simulink model "main_indi"  (R2018a)
settings: Solver=VariableStepAuto  StartTime=0.0  StopTime=inf  RelTol=1e-3
InitFcn:
  | G1_inverse;
undefined symbols (not defined in the file): G1_inv
libraries: aerolibutil x4, shared6dof x1, vrlib x1, simulink x1, powerlib_meascontrol x1, aerolibanimutils x1, aerolibnav x1
settings Model: Creator=PSere  LastModifiedBy=PSere

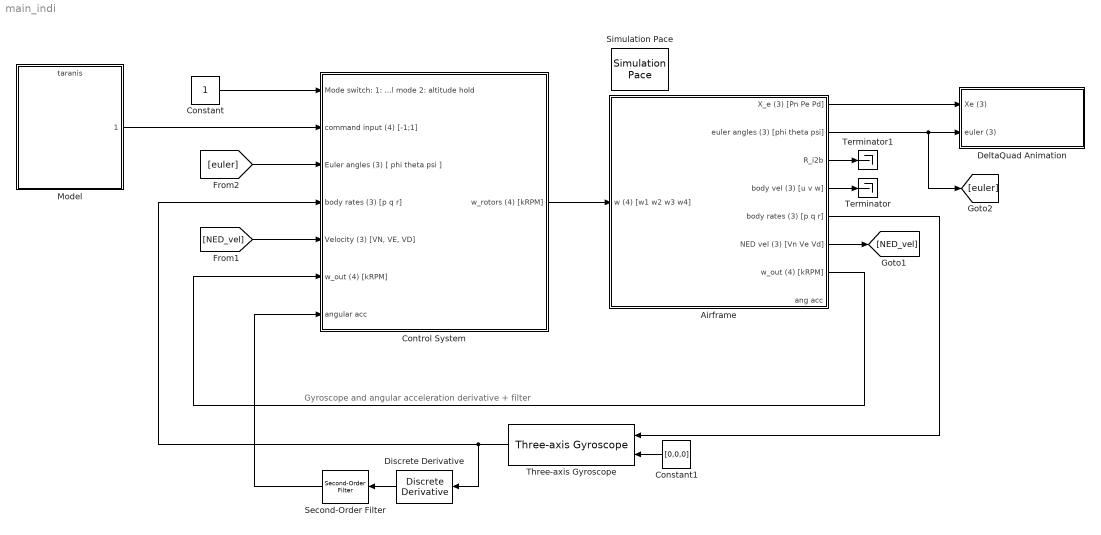
== system main_indi ==
  note: Gyroscope and angular acceleration derivative + filter
  Airframe : Subsystem
  Constant : Constant
  Constant1 : Constant  Value=[0,0,0]
  Control System : Subsystem
  DeltaQuad Animation : Subsystem
  Discrete Derivative : simulink/Discrete/Discrete Derivative  gainval=1.0  ICPrevScaledInput=0.0  OutMin=[]  OutMax=[]  OutDataType=fixdt(1, 16)  OutScaling=2^-10  DoSatur=off
  Model : ModelReference  ModelNameDialog=taranis.mdl  SimulationMode=Normal  ModelReferenceVersion=1.8
  Second-Order Filter : powerlib_meascontrol/Filters/Second-Order Filter  FilterType=Lowpass  Fo=2  Zeta=1  Ts=0  Initialize=on  Vac_Init="[0,  0,  60]"  Vdc_Init=0  PlotResponse=off  FreqRange=[0, 500, 1]
      settings: SourceProductName=Simscape Power Systems  SourceProductBaseCode=PS
  Simulation Pace : aerolibanimutils/Simulation Pace  SimulationPace=1  SleepMode=MATLAB Thread  OutputPaceError=off  SampleTime=1/30
  Terminator : Terminator
  Terminator1 : Terminator
  Three-axis Gyroscope : aerolibnav/Three-axis Gyroscope  dtype_g=on  w_g=190  z_g=0.707  g_sf_cc=[1 0 0; 0 1 0; 0 0 1]  g_bias=[0 0 0]  g_sen=[0 0 0]  g_Ts=0  g_rand=on  g_seeds=[23093 23094 23095]  g_pow=[0.0001 0.0001 0.0001]  g_sat="[-inf  -inf  -inf  inf inf inf]"
      settings: SourceProductName=Aerospace Blockset  SourceProductBaseCode=AE
  wires:
  Model/1 -> Control System/2(command input (4) [-1;1])
  Control System/1(w_rotors (4) [kRPM]) -> Airframe/1(w (4) [w1 w2 w3 w4])
  Airframe/1(X_e (3) [Pn Pe Pd]) -> DeltaQuad Animation/1(Xe (3))
  Airframe/4(body vel (3) [u v w]) -> Terminator/1
  Airframe/2(euler angles (3) [phi theta psi]) -> [euler], DeltaQuad Animation/2(euler (3))
  Airframe/3(R_i2b) -> Terminator1/1
  Constant/1 -> Control System/1(Mode switch: 1: manual mode 2: altitude hold)
  Airframe/5(body rates (3) [p q r]) -> Three-axis Gyroscope/1
  Airframe/6("NED vel (3) [Vn Ve Vd] ") -> [NED_vel]
  [NED_vel] -> Control System/5("Velocity (3) [VN, VE, VD]")
  Three-axis Gyroscope/1 -> Discrete Derivative/1, Control System/4(body rates (3) [p q r])
  [euler] -> Control System/3(Euler angles (3) [ phi theta psi ])
  Airframe/7(w_out (4) [kRPM]) -> Control System/6(w_out (4) [kRPM])
  Constant1/1 -> Three-axis Gyroscope/2
  Discrete Derivative/1 -> Second-Order Filter/1
  Second-Order Filter/1 -> Control System/7(angular acc)

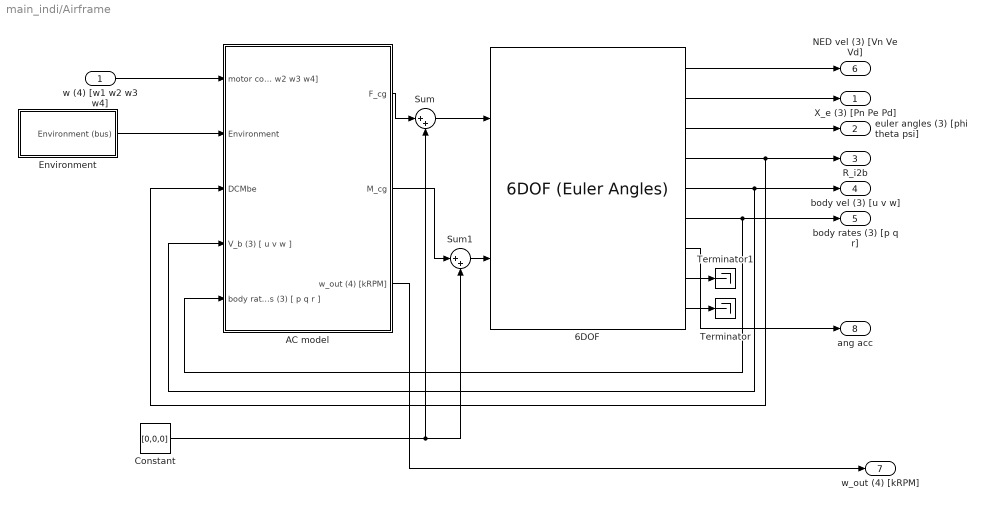
== system main_indi/Airframe ==
  w (4) [w1 w2 w3 w4] : Inport
  6DOF : shared6dof/6DOF (Euler Angles)  units=Metric (MKS)  mtype=Fixed  rep=Euler Angles  xme_0=[0,0,-10]  Vm_0=[0,0,0]  eul_0=[0,0,0]  pm_0=[0,0,0]  mass_0=5.0  mass_e=0.5  mass_f=2.0  inertia=Iv  inertia_e=eye(3)  inertia_f=2*eye(3)  k_quat=Vehicle.SixDOF.quatGain  vre_flag=on  abi_flag=on  aMode=aMode
      settings: SourceProductBaseCode=AE
  AC model : Subsystem
  Constant : Constant  Value=[0,0,0]
  Environment : Subsystem
  Sum : Sum  Inputs=|++
  Sum1 : Sum  Inputs=|++
  Terminator : Terminator
  Terminator1 : Terminator
  X_e (3) [Pn Pe Pd] : Outport
  euler angles (3) [phi theta psi] : Outport  Port=2
  R_i2b : Outport  Port=3
  body vel (3) [u v w] : Outport  Port=4
  body rates (3) [p q r] : Outport  Port=5
  "NED vel (3) [Vn Ve Vd] " : Outport  Port=6
  w_out (4) [kRPM] : Outport  Port=7
  "ang acc " : Outport  Port=8
  wires:
  6DOF/5 -> AC model/4(V_b (3) [ u v w ]), body vel (3) [u v w]/1
  6DOF/9 -> Terminator/1
  6DOF/7 -> "ang acc "/1
  6DOF/1 -> "NED vel (3) [Vn Ve Vd] "/1
  6DOF/6 -> body rates (3) [p q r]/1, AC model/5(body rates (3) [ p q r ])
  Environment/1(Environment (bus)) -> AC model/2(Environment)
  w (4) [w1 w2 w3 w4]/1 -> AC model/1(motor commands (4) [w1 w2 w3 w4])
  AC model/1(F_cg) -> Sum/1
  AC model/2(M_cg) -> Sum1/1
  6DOF/4 -> R_i2b/1, AC model/3(DCMbe)
  6DOF/2 -> X_e (3) [Pn Pe Pd]/1
  6DOF/3 -> euler angles (3) [phi theta psi]/1
  Sum/1 -> 6DOF/1
  Sum1/1 -> 6DOF/2
  Constant/1 -> Sum/2, Sum1/2
  AC model/3(w_out (4) [kRPM]) -> w_out (4) [kRPM]/1
  6DOF/8 -> Terminator1/1

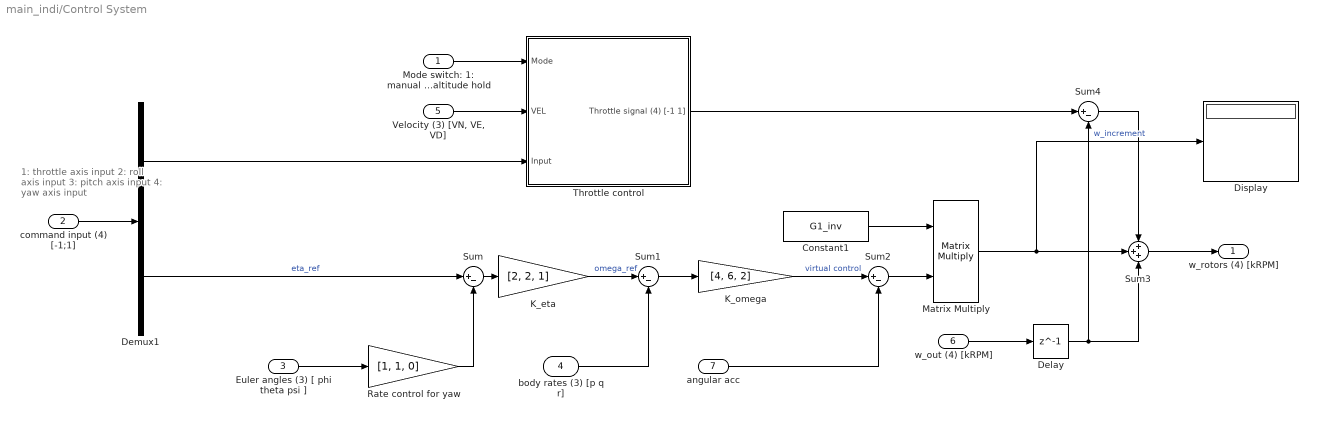
== system main_indi/Control System ==
  note: 1: throttle axis input
      | 2: roll axis input
      | 3: pitch axis input
      | 4: yaw axis input
  Mode switch: 1: manual mode 2: altitude hold : Inport
  command input (4) [-1;1] : Inport  Port=2
  Euler angles (3) [ phi theta psi ] : Inport  Port=3
  body rates (3) [p q r] : Inport  Port=4
  "Velocity (3) [VN, VE, VD]" : Inport  Port=5
  w_out (4) [kRPM] : Inport  Port=6
  angular acc : Inport  Port=7
  Constant1 : Constant  Value=G1_inv
  Delay : Delay  DelayLength=1
  Demux1 : Demux  Outputs=[1 3]
  Display : Display
  K_eta : Gain  Gain=[2, 2, 1]
  K_omega : Gain  Gain=[4, 6, 2]
  Matrix Multiply : Product  Multiplication=Matrix(*)
  Rate control for yaw : Gain  Gain=[1, 1, 0]
  Sum{,1..2,4} (4 alike) : Sum  Inputs=|+-
  Sum3 : Sum  Inputs=+++
  Throttle control : Subsystem
  w_rotors (4) [kRPM] : Outport
  wires:
  command input (4) [-1;1]/1 -> Demux1/1
  Demux1/2 -> Sum/1  "eta_ref"
  Mode switch: 1: manual mode 2: altitude hold/1 -> Throttle control/1(Mode)
  "Velocity (3) [VN, VE, VD]"/1 -> Throttle control/2(VEL)
  Demux1/1 -> Throttle control/3(Input)
  Throttle control/1(Throttle signal (4) [-1 1]) -> Sum4/1
  K_eta/1 -> Sum1/1  "omega_ref"
  Sum/1 -> K_eta/1
  Euler angles (3) [ phi theta psi ]/1 -> Rate control for yaw/1
  body rates (3) [p q r]/1 -> Sum1/2
  Sum1/1 -> K_omega/1
  K_omega/1 -> Sum2/1  "virtual control"
  Sum2/1 -> Matrix Multiply/2
  Constant1/1 -> Matrix Multiply/1
  w_out (4) [kRPM]/1 -> Delay/1
  Sum3/1 -> w_rotors (4) [kRPM]/1
  Delay/1 -> Sum3/3, Sum4/2
  Matrix Multiply/1 -> Display/1, Sum3/2  "w_increment"
  Sum4/1 -> Sum3/1
  Rate control for yaw/1 -> Sum/2
  angular acc/1 -> Sum2/2

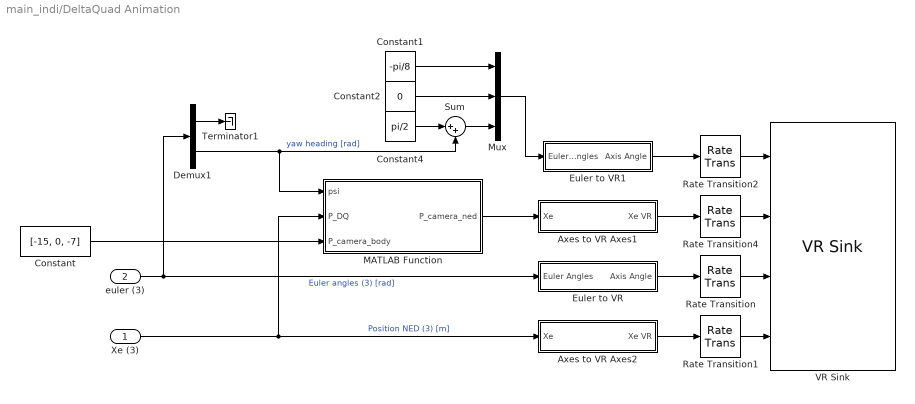
== system main_indi/DeltaQuad Animation ==
  Xe (3) : Inport
  euler (3) : Inport  Port=2
  Axes to VR Axes1 : Subsystem
  Axes to VR Axes2 : Subsystem
  Constant : Constant  Value=[-15, 0, -7]
  Constant1 : Constant  Value=-pi/8
  Constant2 : Constant  Value=0
  Constant4 : Constant  Value=pi/2
  Demux1 : Demux  Outputs=[2 1]
  Euler to VR : Subsystem
  Euler to VR1 : Subsystem
  MATLAB Function : MATLAB Function  TreatAsAtomicUnit=on
  Mux : Mux  Inputs=3
  Rate Transition{,1..2,4} (4 alike) : RateTransition
  Sum : Sum  Inputs=|++
  Terminator1 : Terminator
  VR Sink : vrlib/VR Sink  InstantiateOnLoad=on  SampleTime=-1  ViewEnable=on  RemoteChange=off  RemoteView=off  FieldsWritten=Gimballed.orientation.4.1.1.double#Gimballed.position.3.1.1.double#DeltaQuad.rotation.4.1.1.double#DeltaQuad.translation.3.1.1.double  WorldFileName=animation\DQ_sim_simple.wrl  AutoView=off  VideoDimensions=[]  AllowVariableSize=off
      settings: SourceProductBaseCode=VR
  wires:
  Euler to VR/1(Axis Angle) -> Rate Transition/1
  euler (3)/1 -> Euler to VR/1(Euler Angles), Demux1/1  "Euler angles (3) [rad]"
  Xe (3)/1 -> MATLAB Function/2(P_DQ), Axes to VR Axes2/1(Xe)  "Position NED (3) [m]"
  Axes to VR Axes2/1(Xe VR) -> Rate Transition1/1
  Rate Transition/1 -> VR Sink/3
  Rate Transition1/1 -> VR Sink/4
  Rate Transition4/1 -> VR Sink/2
  Rate Transition2/1 -> VR Sink/1
  Euler to VR1/1(Axis Angle) -> Rate Transition2/1
  Axes to VR Axes1/1(Xe VR) -> Rate Transition4/1
  MATLAB Function/1(P_camera_ned) -> Axes to VR Axes1/1(Xe)
  Constant/1 -> MATLAB Function/3(P_camera_body)
  Sum/1 -> Mux/3
  Demux1/2 -> MATLAB Function/1(psi), Sum/2  "yaw heading [rad]"
  Constant4/1 -> Sum/1
  Constant2/1 -> Mux/2
  Constant1/1 -> Mux/1
  Mux/1 -> Euler to VR1/1(Euler Angles)
  Demux1/1 -> Terminator1/1

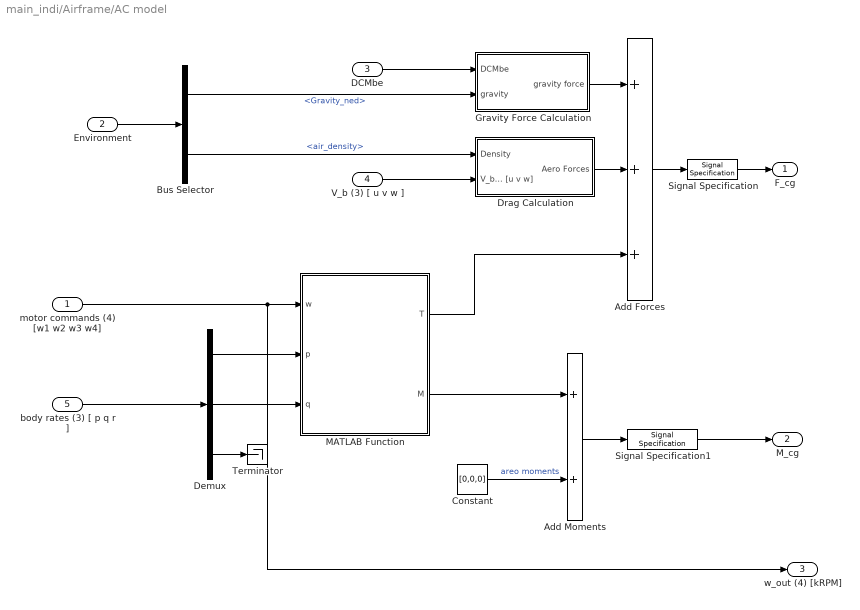
== system main_indi/Airframe/AC model ==
  motor commands (4) [w1 w2 w3 w4] : Inport
  Environment : Inport  Port=2
  DCMbe : Inport  Port=3
  V_b (3) [ u v w ] : Inport  Port=4  Unit=m/s
  body rates (3) [ p q r ] : Inport  Port=5  Unit=rad/s
  Add Forces : Sum  Inputs=+++
  Add Moments : Sum
  Bus Selector : BusSelector  OutputSignals=Gravity_ned,AtmosphereBus.air_density
  Constant : Constant  Value=[0,0,0]
  Demux : Demux  Outputs=3
  Drag Calculation : Subsystem
  Gravity Force Calculation : Subsystem
  MATLAB Function : MATLAB Function  TreatAsAtomicUnit=on
  Signal Specification : SignalSpecification  Dimensions=3
  Signal Specification1 : SignalSpecification  Unit=N*m  Dimensions=3
  Terminator : Terminator
  F_cg : Outport  Unit=N
  M_cg : Outport  Port=2
  w_out (4) [kRPM] : Outport  Port=3
  wires:
  Signal Specification/1 -> F_cg/1
  Bus Selector/1 -> Gravity Force Calculation/2(gravity)  "<Gravity_ned>"
  Environment/1 -> Bus Selector/1
  Bus Selector/2 -> Drag Calculation/1(Density)  "<air_density>"
  DCMbe/1 -> Gravity Force Calculation/1(DCMbe)
  V_b (3) [ u v w ]/1 -> Drag Calculation/2(V_body [u v w])
  Gravity Force Calculation/1(gravity force) -> Add Forces/1
  Drag Calculation/1(Aero Forces) -> Add Forces/2
  Add Forces/1 -> Signal Specification/1
  Add Moments/1 -> Signal Specification1/1
  MATLAB Function/1(T) -> Add Forces/3
  MATLAB Function/2(M) -> Add Moments/1
  Constant/1 -> Add Moments/2  "areo moments"
  Signal Specification1/1 -> M_cg/1
  Demux/2 -> MATLAB Function/3(q)
  Demux/1 -> MATLAB Function/2(p)
  motor commands (4) [w1 w2 w3 w4]/1 -> w_out (4) [kRPM]/1, MATLAB Function/1(w)
  Demux/3 -> Terminator/1
  body rates (3) [ p q r ]/1 -> Demux/1

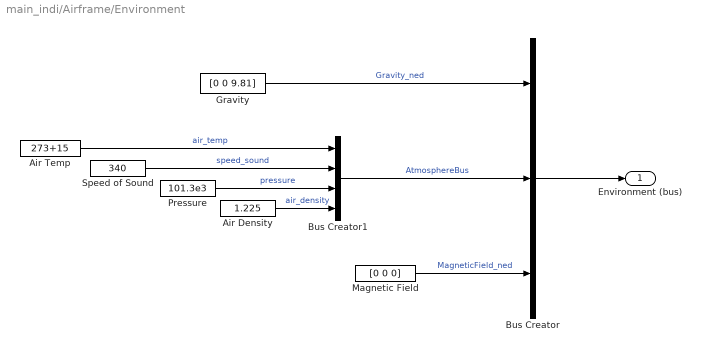
== system main_indi/Airframe/Environment ==
  Air Density : Constant  Value=1.225
  Air Temp : Constant  Value=273+15
  Bus Creator : BusCreator  Inputs=3
  Bus Creator1 : BusCreator  Inputs=4
  Gravity : Constant  Value=[0 0 9.81]
  Magnetic Field : Constant  Value=[0 0 0]
  Pressure : Constant  Value=101.3e3
  Speed of Sound : Constant  Value=340
  Environment (bus) : Outport
  wires:
  Air Temp/1 -> Bus Creator1/1  "air_temp"
  Magnetic Field/1 -> Bus Creator/3  "MagneticField_ned"
  Speed of Sound/1 -> Bus Creator1/2  "speed_sound"
  Gravity/1 -> Bus Creator/1  "Gravity_ned"
  Bus Creator1/1 -> Bus Creator/2  "AtmosphereBus"
  Bus Creator/1 -> Environment (bus)/1
  Air Density/1 -> Bus Creator1/4  "air_density"
  Pressure/1 -> Bus Creator1/3  "pressure"

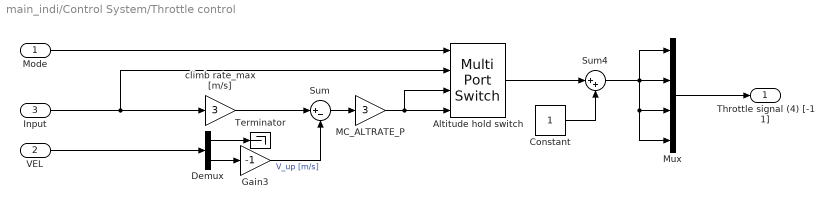
== system main_indi/Control System/Throttle control ==
  Mode : Inport
  VEL : Inport  Port=2
  Input : Inport  Port=3
  Altitude hold switch : MultiPortSwitch
  Constant : Constant
  Demux : Demux  Outputs=[2, 1]
  Gain3 : Gain  Gain=-1
  MC_ALTRATE_P : Gain  Gain=3
  Mux : Mux
  Sum : Sum  Inputs=|+-
  Sum4 : Sum  Inputs=|++
  Terminator : Terminator
  climb rate_max [m/s] : Gain  Gain=3
  Throttle signal (4) [-1 1] : Outport
  wires:
  Sum/1 -> MC_ALTRATE_P/1
  Altitude hold switch/1 -> Sum4/1
  Mode/1 -> Altitude hold switch/1
  Demux/1 -> Terminator/1
  climb rate_max [m/s]/1 -> Sum/1
  Demux/2 -> Gain3/1
  Gain3/1 -> Sum/2  "V_up [m/s]"
  MC_ALTRATE_P/1 -> Altitude hold switch/4, Altitude hold switch/3
  Input/1 -> climb rate_max [m/s]/1, Altitude hold switch/2
  VEL/1 -> Demux/1
  Constant/1 -> Sum4/2
  Sum4/1 -> Mux/4, Mux/3, Mux/1, Mux/2
  Mux/1 -> Throttle signal (4) [-1 1]/1

== system main_indi/DeltaQuad Animation/Axes to VR Axes1 ==
  Xe : Inport
  Demux : Demux  Outputs=3
  Mux : Mux  Inputs=3
  rad-->deg1 : Gain  Gain=-1  SaturateOnIntegerOverflow=on  OutDataTypeStr=Inherit: Same as input  ParamDataTypeStr=Inherit: Same as input
  Xe VR : Outport
  wires:
  Xe/1 -> Demux/1
  Demux/1 -> Mux/1
  Demux/3 -> rad-->deg1/1
  Mux/1 -> Xe VR/1
  rad-->deg1/1 -> Mux/2
  Demux/2 -> Mux/3

== system main_indi/DeltaQuad Animation/Axes to VR Axes2 ==
  Xe : Inport
  Demux : Demux  Outputs=3
  Mux : Mux  Inputs=3
  rad-->deg1 : Gain  Gain=-1  SaturateOnIntegerOverflow=on  OutDataTypeStr=Inherit: Same as input  ParamDataTypeStr=Inherit: Same as input
  Xe VR : Outport
  wires:
  Xe/1 -> Demux/1
  Demux/1 -> Mux/1
  Demux/3 -> rad-->deg1/1
  Mux/1 -> Xe VR/1
  rad-->deg1/1 -> Mux/2
  Demux/2 -> Mux/3

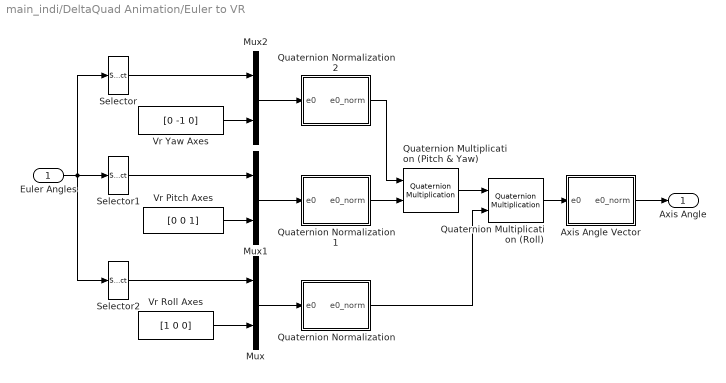
== system main_indi/DeltaQuad Animation/Euler to VR ==
  Euler Angles : Inport
  Axis Angle Vector : Subsystem
  Mux : Mux  Inputs=2
  Mux1 : Mux  Inputs=2
  Mux2 : Mux  Inputs=2
  Quaternion Multiplication (Pitch & Yaw) : aerolibutil/Quaternion Multiplication
  Quaternion Multiplication (Roll) : aerolibutil/Quaternion Multiplication
  Quaternion Normalization : Subsystem
  Quaternion Normalization1 : Subsystem
  Quaternion Normalization2 : Subsystem
  Selector : Selector  InputPortWidth=3  IndexOptions=Index vector (dialog)  Indices=[3]  OutputSizes=1
  Selector1 : Selector  InputPortWidth=3  IndexOptions=Index vector (dialog)  Indices=[2]  OutputSizes=1
  Selector2 : Selector  InputPortWidth=3  IndexOptions=Index vector (dialog)  Indices=[1]  OutputSizes=1
  Vr Pitch Axes : Constant  Value=[0 0 1]
  Vr Roll Axes : Constant  Value=[1 0 0]
  Vr Yaw Axes : Constant  Value=[0 -1 0]
  Axis Angle : Outport
  wires:
  Quaternion Multiplication (Roll)/1 -> Axis Angle Vector/1(e0)
  Axis Angle Vector/1(e0_norm) -> Axis Angle/1
  Quaternion Normalization/1(e0_norm) -> Quaternion Multiplication (Roll)/2
  Quaternion Normalization2/1(e0_norm) -> Quaternion Multiplication (Pitch & Yaw)/1
  Quaternion Normalization1/1(e0_norm) -> Quaternion Multiplication (Pitch & Yaw)/2
  Mux2/1 -> Quaternion Normalization2/1(e0)
  Mux1/1 -> Quaternion Normalization1/1(e0)
  Mux/1 -> Quaternion Normalization/1(e0)
  Selector/1 -> Mux2/1
  Vr Yaw Axes/1 -> Mux2/2
  Selector1/1 -> Mux1/1
  Vr Pitch Axes/1 -> Mux1/2
  Selector2/1 -> Mux/1
  Vr Roll Axes/1 -> Mux/2
  Euler Angles/1 -> Selector2/1, Selector1/1, Selector/1
  Quaternion Multiplication (Pitch & Yaw)/1 -> Quaternion Multiplication (Roll)/1

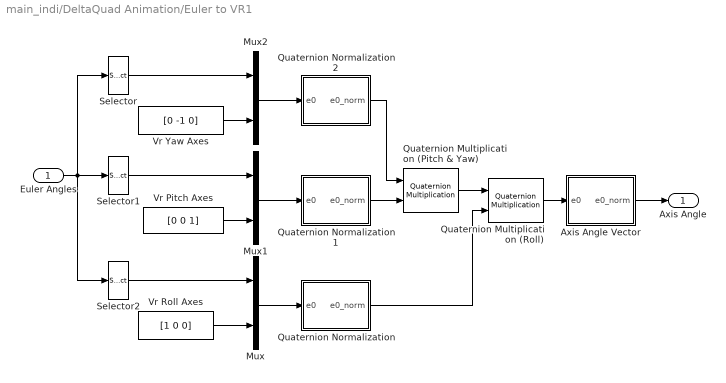
== system main_indi/DeltaQuad Animation/Euler to VR1 ==
  Euler Angles : Inport
  Axis Angle Vector : Subsystem
  Mux : Mux  Inputs=2
  Mux1 : Mux  Inputs=2
  Mux2 : Mux  Inputs=2
  Quaternion Multiplication (Pitch & Yaw) : aerolibutil/Quaternion Multiplication
  Quaternion Multiplication (Roll) : aerolibutil/Quaternion Multiplication
  Quaternion Normalization : Subsystem
  Quaternion Normalization1 : Subsystem
  Quaternion Normalization2 : Subsystem
  Selector : Selector  InputPortWidth=3  IndexOptions=Index vector (dialog)  Indices=[3]  OutputSizes=1
  Selector1 : Selector  InputPortWidth=3  IndexOptions=Index vector (dialog)  Indices=[2]  OutputSizes=1
  Selector2 : Selector  InputPortWidth=3  IndexOptions=Index vector (dialog)  Indices=[1]  OutputSizes=1
  Vr Pitch Axes : Constant  Value=[0 0 1]
  Vr Roll Axes : Constant  Value=[1 0 0]
  Vr Yaw Axes : Constant  Value=[0 -1 0]
  Axis Angle : Outport
  wires:
  Quaternion Multiplication (Roll)/1 -> Axis Angle Vector/1(e0)
  Axis Angle Vector/1(e0_norm) -> Axis Angle/1
  Quaternion Normalization/1(e0_norm) -> Quaternion Multiplication (Roll)/2
  Quaternion Normalization2/1(e0_norm) -> Quaternion Multiplication (Pitch & Yaw)/1
  Quaternion Normalization1/1(e0_norm) -> Quaternion Multiplication (Pitch & Yaw)/2
  Mux2/1 -> Quaternion Normalization2/1(e0)
  Mux1/1 -> Quaternion Normalization1/1(e0)
  Mux/1 -> Quaternion Normalization/1(e0)
  Selector/1 -> Mux2/1
  Vr Yaw Axes/1 -> Mux2/2
  Selector1/1 -> Mux1/1
  Vr Pitch Axes/1 -> Mux1/2
  Selector2/1 -> Mux/1
  Vr Roll Axes/1 -> Mux/2
  Euler Angles/1 -> Selector2/1, Selector1/1, Selector/1
  Quaternion Multiplication (Pitch & Yaw)/1 -> Quaternion Multiplication (Roll)/1

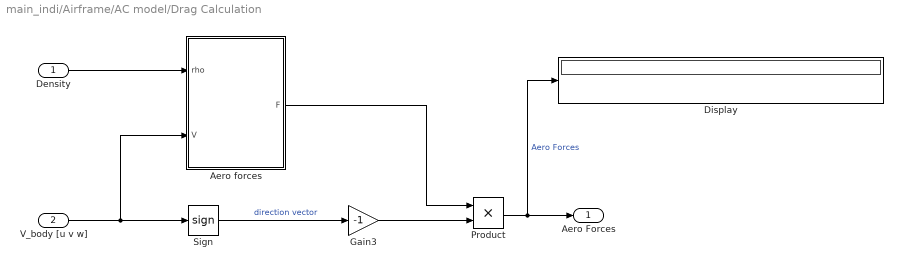
== system main_indi/Airframe/AC model/Drag Calculation ==
  Density : Inport  Unit=kg/m^3
  V_body [u v w] : Inport  Port=2  Unit=m/second
  Aero forces : MATLAB Function  TreatAsAtomicUnit=on
  Display : Display
  Gain3 : Gain  Gain=-1
  Product : Product  RndMeth=Zero
  Sign : Signum  ZeroCross=off
  Aero Forces : Outport  Unit=N
  wires:
  Sign/1 -> Gain3/1  "direction vector"
  Gain3/1 -> Product/2
  Product/1 -> Display/1, Aero Forces/1  "Aero Forces"
  V_body [u v w]/1 -> Aero forces/2(V), Sign/1
  Density/1 -> Aero forces/1(rho)
  Aero forces/1(F) -> Product/1

== system main_indi/Airframe/AC model/Gravity Force Calculation ==
  DCMbe : Inport
  gravity : Inport  Port=2  Unit=m/s^2
  Gain1 : Gain  Gain=5.0
  Product : Product  Multiplication=Matrix(*)
  gravity force : Outport  Unit=N
  wires:
  gravity/1 -> Gain1/1
  Gain1/1 -> Product/2  "gravity force NED"
  Product/1 -> gravity force/1
  DCMbe/1 -> Product/1

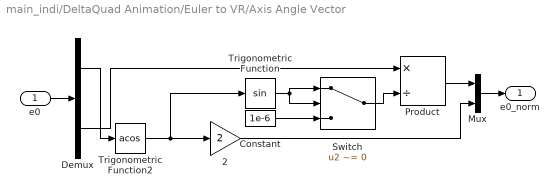
== system main_indi/DeltaQuad Animation/Euler to VR/Axis Angle Vector ==
  e0 : Inport
  2 : Gain  Gain=2  SaturateOnIntegerOverflow=on  OutDataTypeStr=Inherit: Same as input  ParamDataTypeStr=Inherit: Same as input
  Constant : Constant  Value=1e-6
  Demux : Demux  Outputs=[1 3 ]
  Mux : Mux  Inputs=2
  Product : Product  Inputs=*/  SaturateOnIntegerOverflow=on  InputSameDT=on  OutDataTypeStr=Inherit: Same as first input
  Switch : Switch  Criteria=u2 ~= 0
  Trigonometric Function : Trigonometry
  Trigonometric Function2 : Trigonometry  Operator=acos
  e0_norm : Outport
  wires:
  Demux/1 -> Trigonometric Function2/1
  Demux/2 -> Product/1
  Mux/1 -> e0_norm/1
  Product/1 -> Mux/1
  2/1 -> Mux/2
  Trigonometric Function/1 -> Switch/1, Switch/2
  Trigonometric Function2/1 -> Trigonometric Function/1, 2/1
  e0/1 -> Demux/1
  Constant/1 -> Switch/3
  Switch/1 -> Product/2

== system main_indi/DeltaQuad Animation/Euler to VR/Quaternion Normalization ==
  e0 : Inport
  1/2 : Gain  Gain=1/2  SaturateOnIntegerOverflow=on  OutDataTypeStr=Inherit: Same as input  ParamDataTypeStr=Inherit: Same as input
  Demux : Demux  Outputs=[1 3]
  Mux : Mux  Inputs=2
  Product : Product  SaturateOnIntegerOverflow=on  InputSameDT=on  OutDataTypeStr=Inherit: Same as first input
  Trigonometric Function : Trigonometry
  Trigonometric Function1 : Trigonometry  Operator=cos
  e0_norm : Outport
  wires:
  Trigonometric Function1/1 -> Mux/1
  Demux/2 -> Product/2
  Demux/1 -> 1/2/1
  Mux/1 -> e0_norm/1
  Product/1 -> Mux/2
  Trigonometric Function/1 -> Product/1
  1/2/1 -> Trigonometric Function1/1, Trigonometric Function/1
  e0/1 -> Demux/1

== system main_indi/DeltaQuad Animation/Euler to VR/Quaternion Normalization1 ==
  e0 : Inport
  1/2 : Gain  Gain=1/2  SaturateOnIntegerOverflow=on  OutDataTypeStr=Inherit: Same as input  ParamDataTypeStr=Inherit: Same as input
  Demux : Demux  Outputs=[1 3]
  Mux : Mux  Inputs=2
  Product : Product  SaturateOnIntegerOverflow=on  InputSameDT=on  OutDataTypeStr=Inherit: Same as first input
  Trigonometric Function : Trigonometry
  Trigonometric Function1 : Trigonometry  Operator=cos
  e0_norm : Outport
  wires:
  e0/1 -> Demux/1
  1/2/1 -> Trigonometric Function/1, Trigonometric Function1/1
  Trigonometric Function/1 -> Product/1
  Product/1 -> Mux/2
  Mux/1 -> e0_norm/1
  Demux/1 -> 1/2/1
  Demux/2 -> Product/2
  Trigonometric Function1/1 -> Mux/1

== system main_indi/DeltaQuad Animation/Euler to VR/Quaternion Normalization2 ==
  e0 : Inport
  1/2 : Gain  Gain=1/2  SaturateOnIntegerOverflow=on  OutDataTypeStr=Inherit: Same as input  ParamDataTypeStr=Inherit: Same as input
  Demux : Demux  Outputs=[1 3]
  Mux : Mux  Inputs=2
  Product : Product  SaturateOnIntegerOverflow=on  InputSameDT=on  OutDataTypeStr=Inherit: Same as first input
  Trigonometric Function : Trigonometry
  Trigonometric Function1 : Trigonometry  Operator=cos
  e0_norm : Outport
  wires:
  Trigonometric Function1/1 -> Mux/1
  Demux/2 -> Product/2
  Demux/1 -> 1/2/1
  Mux/1 -> e0_norm/1
  Product/1 -> Mux/2
  Trigonometric Function/1 -> Product/1
  1/2/1 -> Trigonometric Function1/1, Trigonometric Function/1
  e0/1 -> Demux/1

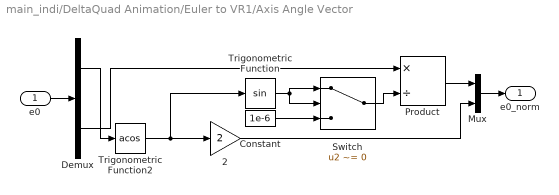
== system main_indi/DeltaQuad Animation/Euler to VR1/Axis Angle Vector ==
  e0 : Inport
  2 : Gain  Gain=2  SaturateOnIntegerOverflow=on  OutDataTypeStr=Inherit: Same as input  ParamDataTypeStr=Inherit: Same as input
  Constant : Constant  Value=1e-6
  Demux : Demux  Outputs=[1 3 ]
  Mux : Mux  Inputs=2
  Product : Product  Inputs=*/  SaturateOnIntegerOverflow=on  InputSameDT=on  OutDataTypeStr=Inherit: Same as first input
  Switch : Switch  Criteria=u2 ~= 0
  Trigonometric Function : Trigonometry
  Trigonometric Function2 : Trigonometry  Operator=acos
  e0_norm : Outport
  wires:
  Demux/1 -> Trigonometric Function2/1
  Demux/2 -> Product/1
  Mux/1 -> e0_norm/1
  Product/1 -> Mux/1
  2/1 -> Mux/2
  Trigonometric Function/1 -> Switch/1, Switch/2
  Trigonometric Function2/1 -> Trigonometric Function/1, 2/1
  e0/1 -> Demux/1
  Constant/1 -> Switch/3
  Switch/1 -> Product/2

== system main_indi/DeltaQuad Animation/Euler to VR1/Quaternion Normalization ==
  e0 : Inport
  1/2 : Gain  Gain=1/2  SaturateOnIntegerOverflow=on  OutDataTypeStr=Inherit: Same as input  ParamDataTypeStr=Inherit: Same as input
  Demux : Demux  Outputs=[1 3]
  Mux : Mux  Inputs=2
  Product : Product  SaturateOnIntegerOverflow=on  InputSameDT=on  OutDataTypeStr=Inherit: Same as first input
  Trigonometric Function : Trigonometry
  Trigonometric Function1 : Trigonometry  Operator=cos
  e0_norm : Outport
  wires:
  Trigonometric Function1/1 -> Mux/1
  Demux/2 -> Product/2
  Demux/1 -> 1/2/1
  Mux/1 -> e0_norm/1
  Product/1 -> Mux/2
  Trigonometric Function/1 -> Product/1
  1/2/1 -> Trigonometric Function1/1, Trigonometric Function/1
  e0/1 -> Demux/1

== system main_indi/DeltaQuad Animation/Euler to VR1/Quaternion Normalization1 ==
  e0 : Inport
  1/2 : Gain  Gain=1/2  SaturateOnIntegerOverflow=on  OutDataTypeStr=Inherit: Same as input  ParamDataTypeStr=Inherit: Same as input
  Demux : Demux  Outputs=[1 3]
  Mux : Mux  Inputs=2
  Product : Product  SaturateOnIntegerOverflow=on  InputSameDT=on  OutDataTypeStr=Inherit: Same as first input
  Trigonometric Function : Trigonometry
  Trigonometric Function1 : Trigonometry  Operator=cos
  e0_norm : Outport
  wires:
  e0/1 -> Demux/1
  1/2/1 -> Trigonometric Function/1, Trigonometric Function1/1
  Trigonometric Function/1 -> Product/1
  Product/1 -> Mux/2
  Mux/1 -> e0_norm/1
  Demux/1 -> 1/2/1
  Demux/2 -> Product/2
  Trigonometric Function1/1 -> Mux/1

== system main_indi/DeltaQuad Animation/Euler to VR1/Quaternion Normalization2 ==
  e0 : Inport
  1/2 : Gain  Gain=1/2  SaturateOnIntegerOverflow=on  OutDataTypeStr=Inherit: Same as input  ParamDataTypeStr=Inherit: Same as input
  Demux : Demux  Outputs=[1 3]
  Mux : Mux  Inputs=2
  Product : Product  SaturateOnIntegerOverflow=on  InputSameDT=on  OutDataTypeStr=Inherit: Same as first input
  Trigonometric Function : Trigonometry
  Trigonometric Function1 : Trigonometry  Operator=cos
  e0_norm : Outport
  wires:
  Trigonometric Function1/1 -> Mux/1
  Demux/2 -> Product/2
  Demux/1 -> 1/2/1
  Mux/1 -> e0_norm/1
  Product/1 -> Mux/2
  Trigonometric Function/1 -> Product/1
  1/2/1 -> Trigonometric Function1/1, Trigonometric Function/1
  e0/1 -> Demux/1

== matlab function main_indi/Airframe/AC model/Drag Calculation/Aero forces ==
  data: rho input; V input; F output
function F = aero(rho, V)
%% INPUTS:
% rho:  density                              [kg/m3]
% V:    body velocities wrt air [ub, vb, wb] [m/s]
%TAS = norm(V);
%alpha = atan(V(3)/V(1));

%% DQ Parameters:
%S = 1.0;
%b = 1.9;

%e = 0.9;
%AR = b^2/S;
%qS = 0.5*rho*TAS^2*S;

%% Aerodynamic coefficients:
%Within 20 degree region we generate lift:
% 
% CL_0        = 0.0;
% CD_0        = 0.02;
% if abs(alpha*180/pi) < 10
%     CL_alpha = 1.1471;
%     
%     CL = CL_0 + CL_alpha * alpha;
%     CD = CD_0 + CL^2 / (pi*AR*e);
%     CY = 0;
%     
%     % Rotate the coordinate frame around Y-axis with alpha to get body axes 
%     F_liftdrag = [cos(alpha)    0   -sin(alpha);
%                   0             1   0;
%                   sin(alpha)    0   cos(alpha)]*[qS * CD; 
%                                                  qS * CY; 
%                                                  qS * CL];
%                                              
%                  
% else
% 
%     F_liftdrag = [0;0;0];
% end

F_liftdrag = [0;0;0];

S = 1.0;

CD_X = 0.1;
CD_Y = 0.1;
CD_Z = 0.2;

F = [0.5 * rho * S * V(1)^2 * CD_X;
     0.5 * rho * S * V(2)^2 * CD_Y;
     0.5 * rho * S * V(3)^2 * CD_Z] + F_liftdrag;



end

% Moments:
% %% Roll pitch and yaw moments as a function of alpha and beta:
% 
% Cl = Cl_beta  * beta;
% Cm = Cm_0 + Cm_alpha * alpha;
% Cn = Cn_beta  * beta;
% 
% Ma = [  b * qS * Cl; 
%         c * qS * Cm; 
%         b * qS * Cn];

== matlab function main_indi/Airframe/AC model/MATLAB Function ==
  data: w input; T output; M output; p input; q input
function [T, M] = motor_model(w, p, q)
%% Deltaquad Parameters:
      
Irzz    = 0.05;                            % rotor inertia [kgm2]
dx      = 0.35;                            % position of rotors x
dy      = 0.35;                            % position of rotors y
k1      = 12.2625;                         % N / kRPM^2
k2      = 4.2;                             % Nm / kRPM^2

if length(w) ~= 4
    error('control vector wrong size')
end

%% Thrust and Moments:
% 1) Total Thrust body axis
T = [0; 0; -k1 * sum(w.^2)];

% 2) Mc: Conrol moments:
Mc = [-dy*k1, dy*k1,  dy*k1, -dy*k1;
       dx*k1, dx*k1, -dx*k1, -dx*k1;
       k2,    -k2,    k2,      -k2]*w.^2;
   
% 3) Mr: Gyroscopic effect:
Mr = [ Irzz*q, -Irzz*q,  Irzz*q, -Irzz*q;
      -Irzz*p,  Irzz*p, -Irzz*p,  Irzz*p;
            0,       0,       0,       0]*w;

M = Mc - Mr;

== matlab function main_indi/DeltaQuad Animation/MATLAB Function ==
  data: psi input; P_DQ input; P_camera_ned output; P_camera_body input
function P_camera_ned  = fcn(psi, P_DQ, P_camera_body)
R_b2i_phi = transpose([cos(psi), sin(psi),    0; -sin(psi), cos(psi),   0; 0, 0, 1]);
P_camera_ned = [P_DQ(1);P_DQ(2);P_DQ(3)] + R_b2i_phi * [P_camera_body(1);P_camera_body(2);P_camera_body(3)];
